simulink model "cpg_optimized"  (R2016a)
settings: Solver=FixedStepAuto  StartTime=0.0  StopTime=inf  FixedStep=0.04  RelTol=1e-3
values from neighbouring files (symbols this model uses):
  A_f = 0.1    [setup.m]
  ICNotPresent = 1    [setup.m]
  joints_in_use = [j_i_m('l_leg_hpx') j_i_m('l_leg_hpy') j_i_m('l_leg_kny') j_i_m('l_leg_aky') j_i_m('l_leg_akx') j_i_m('l_arm_shx') j_i_m('r_leg_hpx') j_i_m('r_leg_hpy') j_i_m('r_leg_kny') j_i_m('r_leg_aky') j_i_m('r_leg_akx') j_i_m('r_arm_shx')]    [setup.m]
  sigma_f = 2.2    [setup.m]
  sigma_s = 1    [setup.m]
  t_m = 0.1    [setup.m]
  t_s = 2    [setup.m]
undefined symbols (not defined in the file or in its folder): DiscIntNeverNeededParam, get, Position, SendJointCommand, SetThisJoint
libraries: fuzblock x72, dspsnks4 x4, simulink x2, robotlib x2, dspsrcs4 x1, dspindex x1, sldrtlib x1
(part 2 of 2)

== system cpg_optimized/cell_18_2 ==
  In1 : Inport
  Add : Sum  Inputs=++-
  Add1 : Sum  Inputs=-+
  Add2 : Sum  Inputs=-+
  DTI_1 : DiscreteIntegrator  InitialCondition=0.065208  InitialConditionSetting=State (most efficient)  SampleTime=-1  ICPrevOutput=DiscIntNeverNeededParam  ICPrevScaledInput=DiscIntNeverNeededParam
  DTI_2 : DiscreteIntegrator  InitialCondition=0.029689  InitialConditionSetting=State (most efficient)  SampleTime=-1  ICPrevOutput=DiscIntNeverNeededParam  ICPrevScaledInput=DiscIntNeverNeededParam
  Gain : Gain  Gain=-1/t_m
  Gain1 : Gain  Gain=1/t_s
  Gain2 : Gain  Gain=sigma_s
  Gain3 : Gain  Gain=A_f
  Gain4 : Gain  Gain=sigma_f/A_f
  Trigonometric Function : Trigonometry  Operator=tanh
  Out1 : Outport
  wires:
  Gain/1 -> DTI_1/1
  Add/1 -> Gain/1
  Gain2/1 -> Add1/2
  Gain3/1 -> Add2/1
  Add2/1 -> Add/1
  DTI_1/1 -> Out1/1, Gain2/1, Gain4/1, Add2/2  "V"
  Trigonometric Function/1 -> Gain3/1
  Gain4/1 -> Trigonometric Function/1
  In1/1 -> Add/3
  Add1/1 -> Gain1/1
  Gain1/1 -> DTI_2/1
  DTI_2/1 -> Add1/1, Add/2  "q"

== system cpg_optimized/cell_25_1 ==
  In1 : Inport
  Add : Sum  Inputs=++-
  Add1 : Sum  Inputs=-+
  Add2 : Sum  Inputs=-+
  DTI_1 : DiscreteIntegrator  InitialCondition=0.065208  InitialConditionSetting=State (most efficient)  SampleTime=-1  ICPrevOutput=DiscIntNeverNeededParam  ICPrevScaledInput=DiscIntNeverNeededParam
  DTI_2 : DiscreteIntegrator  InitialCondition=0.029689  InitialConditionSetting=State (most efficient)  SampleTime=-1  ICPrevOutput=DiscIntNeverNeededParam  ICPrevScaledInput=DiscIntNeverNeededParam
  Gain : Gain  Gain=-1/t_m
  Gain1 : Gain  Gain=1/t_s
  Gain2 : Gain  Gain=sigma_s
  Gain3 : Gain  Gain=A_f
  Gain4 : Gain  Gain=sigma_f/A_f
  Trigonometric Function : Trigonometry  Operator=tanh
  Out1 : Outport
  wires:
  Gain/1 -> DTI_1/1
  Add/1 -> Gain/1
  Gain2/1 -> Add1/2
  Gain3/1 -> Add2/1
  Add2/1 -> Add/1
  DTI_1/1 -> Out1/1, Gain2/1, Gain4/1, Add2/2  "V"
  Trigonometric Function/1 -> Gain3/1
  Gain4/1 -> Trigonometric Function/1
  In1/1 -> Add/3
  Add1/1 -> Gain1/1
  Gain1/1 -> DTI_2/1
  DTI_2/1 -> Add1/1, Add/2  "q"

== system cpg_optimized/cell_25_2 ==
  In1 : Inport
  Add : Sum  Inputs=++-
  Add1 : Sum  Inputs=-+
  Add2 : Sum  Inputs=-+
  DTI_1 : DiscreteIntegrator  InitialCondition=-0.065208  InitialConditionSetting=State (most efficient)  SampleTime=-1  ICPrevOutput=DiscIntNeverNeededParam  ICPrevScaledInput=DiscIntNeverNeededParam
  DTI_2 : DiscreteIntegrator  InitialCondition=-0.029689  InitialConditionSetting=State (most efficient)  SampleTime=-1  ICPrevOutput=DiscIntNeverNeededParam  ICPrevScaledInput=DiscIntNeverNeededParam
  Gain : Gain  Gain=-1/t_m
  Gain1 : Gain  Gain=1/t_s
  Gain2 : Gain  Gain=sigma_s
  Gain3 : Gain  Gain=A_f
  Gain4 : Gain  Gain=sigma_f/A_f
  Trigonometric Function : Trigonometry  Operator=tanh
  Out1 : Outport
  wires:
  Gain/1 -> DTI_1/1
  Add/1 -> Gain/1
  Gain2/1 -> Add1/2
  Gain3/1 -> Add2/1
  Add2/1 -> Add/1
  DTI_1/1 -> Out1/1, Gain2/1, Gain4/1, Add2/2  "V"
  Trigonometric Function/1 -> Gain3/1
  Gain4/1 -> Trigonometric Function/1
  In1/1 -> Add/3
  Add1/1 -> Gain1/1
  Gain1/1 -> DTI_2/1
  DTI_2/1 -> Add1/1, Add/2  "q"

== system cpg_optimized/cell_6_1 ==
  In1 : Inport
  Add : Sum  Inputs=++-
  Add1 : Sum  Inputs=-+
  Add2 : Sum  Inputs=-+
  DTI_1 : DiscreteIntegrator  InitialCondition=-0.059359  InitialConditionSetting=State (most efficient)  SampleTime=-1  ICPrevOutput=DiscIntNeverNeededParam  ICPrevScaledInput=DiscIntNeverNeededParam
  DTI_2 : DiscreteIntegrator  InitialCondition=-0.031714  InitialConditionSetting=State (most efficient)  SampleTime=-1  ICPrevOutput=DiscIntNeverNeededParam  ICPrevScaledInput=DiscIntNeverNeededParam
  Gain : Gain  Gain=-1/t_m
  Gain1 : Gain  Gain=1/t_s
  Gain2 : Gain  Gain=sigma_s
  Gain3 : Gain  Gain=A_f
  Gain4 : Gain  Gain=sigma_f/A_f
  Trigonometric Function : Trigonometry  Operator=tanh
  Out1 : Outport
  wires:
  Gain/1 -> DTI_1/1
  Add/1 -> Gain/1
  Gain2/1 -> Add1/2
  Gain3/1 -> Add2/1
  Add2/1 -> Add/1
  DTI_1/1 -> Out1/1, Gain2/1, Gain4/1, Add2/2  "V"
  Trigonometric Function/1 -> Gain3/1
  Gain4/1 -> Trigonometric Function/1
  In1/1 -> Add/3
  Add1/1 -> Gain1/1
  Gain1/1 -> DTI_2/1
  DTI_2/1 -> Add1/1, Add/2  "q"

== system cpg_optimized/cell_6_2 ==
  In1 : Inport
  Add : Sum  Inputs=++-
  Add1 : Sum  Inputs=-+
  Add2 : Sum  Inputs=-+
  DTI_1 : DiscreteIntegrator  InitialCondition=0.059359  InitialConditionSetting=State (most efficient)  SampleTime=-1  ICPrevOutput=DiscIntNeverNeededParam  ICPrevScaledInput=DiscIntNeverNeededParam
  DTI_2 : DiscreteIntegrator  InitialCondition=0.031714  InitialConditionSetting=State (most efficient)  SampleTime=-1  ICPrevOutput=DiscIntNeverNeededParam  ICPrevScaledInput=DiscIntNeverNeededParam
  Gain : Gain  Gain=-1/t_m
  Gain1 : Gain  Gain=1/t_s
  Gain2 : Gain  Gain=sigma_s
  Gain3 : Gain  Gain=A_f
  Gain4 : Gain  Gain=sigma_f/A_f
  Trigonometric Function : Trigonometry  Operator=tanh
  Out1 : Outport
  wires:
  Gain/1 -> DTI_1/1
  Add/1 -> Gain/1
  Gain2/1 -> Add1/2
  Gain3/1 -> Add2/1
  Add2/1 -> Add/1
  DTI_1/1 -> Out1/1, Gain2/1, Gain4/1, Add2/2  "V"
  Trigonometric Function/1 -> Gain3/1
  Gain4/1 -> Trigonometric Function/1
  In1/1 -> Add/3
  Add1/1 -> Gain1/1
  Gain1/1 -> DTI_2/1
  DTI_2/1 -> Add1/1, Add/2  "q"

== system cpg_optimized/cell_7_1 ==
  In1 : Inport
  Add : Sum  Inputs=++-
  Add1 : Sum  Inputs=-+
  Add2 : Sum  Inputs=-+
  DTI_1 : DiscreteIntegrator  InitialCondition=0.059359  InitialConditionSetting=State (most efficient)  SampleTime=-1  ICPrevOutput=DiscIntNeverNeededParam  ICPrevScaledInput=DiscIntNeverNeededParam
  DTI_2 : DiscreteIntegrator  InitialCondition=0.031714  InitialConditionSetting=State (most efficient)  SampleTime=-1  ICPrevOutput=DiscIntNeverNeededParam  ICPrevScaledInput=DiscIntNeverNeededParam
  Gain : Gain  Gain=-1/t_m
  Gain1 : Gain  Gain=1/t_s
  Gain2 : Gain  Gain=sigma_s
  Gain3 : Gain  Gain=A_f
  Gain4 : Gain  Gain=sigma_f/A_f
  Trigonometric Function : Trigonometry  Operator=tanh
  Out1 : Outport
  wires:
  Gain/1 -> DTI_1/1
  Add/1 -> Gain/1
  Gain2/1 -> Add1/2
  Gain3/1 -> Add2/1
  Add2/1 -> Add/1
  DTI_1/1 -> Out1/1, Gain2/1, Gain4/1, Add2/2  "V"
  Trigonometric Function/1 -> Gain3/1
  Gain4/1 -> Trigonometric Function/1
  In1/1 -> Add/3
  Add1/1 -> Gain1/1
  Gain1/1 -> DTI_2/1
  DTI_2/1 -> Add1/1, Add/2  "q"

== system cpg_optimized/cell_7_2 ==
  In1 : Inport
  Add : Sum  Inputs=++-
  Add1 : Sum  Inputs=-+
  Add2 : Sum  Inputs=-+
  DTI_1 : DiscreteIntegrator  InitialCondition=-0.059359  InitialConditionSetting=State (most efficient)  SampleTime=-1  ICPrevOutput=DiscIntNeverNeededParam  ICPrevScaledInput=DiscIntNeverNeededParam
  DTI_2 : DiscreteIntegrator  InitialCondition=-0.031714  InitialConditionSetting=State (most efficient)  SampleTime=-1  ICPrevOutput=DiscIntNeverNeededParam  ICPrevScaledInput=DiscIntNeverNeededParam
  Gain : Gain  Gain=-1/t_m
  Gain1 : Gain  Gain=1/t_s
  Gain2 : Gain  Gain=sigma_s
  Gain3 : Gain  Gain=A_f
  Gain4 : Gain  Gain=sigma_f/A_f
  Trigonometric Function : Trigonometry  Operator=tanh
  Out1 : Outport
  wires:
  Gain/1 -> DTI_1/1
  Add/1 -> Gain/1
  Gain2/1 -> Add1/2
  Gain3/1 -> Add2/1
  Add2/1 -> Add/1
  DTI_1/1 -> Out1/1, Gain2/1, Gain4/1, Add2/2  "V"
  Trigonometric Function/1 -> Gain3/1
  Gain4/1 -> Trigonometric Function/1
  In1/1 -> Add/3
  Add1/1 -> Gain1/1
  Gain1/1 -> DTI_2/1
  DTI_2/1 -> Add1/1, Add/2  "q"

== system cpg_optimized/cell_8_1 ==
  In1 : Inport
  Add : Sum  Inputs=++-
  Add1 : Sum  Inputs=-+
  Add2 : Sum  Inputs=-+
  DTI_1 : DiscreteIntegrator  InitialCondition=0.059359  InitialConditionSetting=State (most efficient)  SampleTime=-1  ICPrevOutput=DiscIntNeverNeededParam  ICPrevScaledInput=DiscIntNeverNeededParam
  DTI_2 : DiscreteIntegrator  InitialCondition=0.031714  InitialConditionSetting=State (most efficient)  SampleTime=-1  ICPrevOutput=DiscIntNeverNeededParam  ICPrevScaledInput=DiscIntNeverNeededParam
  Gain : Gain  Gain=-1/t_m
  Gain1 : Gain  Gain=1/t_s
  Gain2 : Gain  Gain=sigma_s
  Gain3 : Gain  Gain=A_f
  Gain4 : Gain  Gain=sigma_f/A_f
  Trigonometric Function : Trigonometry  Operator=tanh
  Out1 : Outport
  wires:
  Gain/1 -> DTI_1/1
  Add/1 -> Gain/1
  Gain2/1 -> Add1/2
  Gain3/1 -> Add2/1
  Add2/1 -> Add/1
  DTI_1/1 -> Out1/1, Gain2/1, Gain4/1, Add2/2  "V"
  Trigonometric Function/1 -> Gain3/1
  Gain4/1 -> Trigonometric Function/1
  In1/1 -> Add/3
  Add1/1 -> Gain1/1
  Gain1/1 -> DTI_2/1
  DTI_2/1 -> Add1/1, Add/2  "q"

== system cpg_optimized/cell_8_2 ==
  In1 : Inport
  Add : Sum  Inputs=++-
  Add1 : Sum  Inputs=-+
  Add2 : Sum  Inputs=-+
  DTI_1 : DiscreteIntegrator  InitialCondition=-0.059359  InitialConditionSetting=State (most efficient)  SampleTime=-1  ICPrevOutput=DiscIntNeverNeededParam  ICPrevScaledInput=DiscIntNeverNeededParam
  DTI_2 : DiscreteIntegrator  InitialCondition=-0.031714  InitialConditionSetting=State (most efficient)  SampleTime=-1  ICPrevOutput=DiscIntNeverNeededParam  ICPrevScaledInput=DiscIntNeverNeededParam
  Gain : Gain  Gain=-1/t_m
  Gain1 : Gain  Gain=1/t_s
  Gain2 : Gain  Gain=sigma_s
  Gain3 : Gain  Gain=A_f
  Gain4 : Gain  Gain=sigma_f/A_f
  Trigonometric Function : Trigonometry  Operator=tanh
  Out1 : Outport
  wires:
  Gain/1 -> DTI_1/1
  Add/1 -> Gain/1
  Gain2/1 -> Add1/2
  Gain3/1 -> Add2/1
  Add2/1 -> Add/1
  DTI_1/1 -> Out1/1, Gain2/1, Gain4/1, Add2/2  "V"
  Trigonometric Function/1 -> Gain3/1
  Gain4/1 -> Trigonometric Function/1
  In1/1 -> Add/3
  Add1/1 -> Gain1/1
  Gain1/1 -> DTI_2/1
  DTI_2/1 -> Add1/1, Add/2  "q"

== system cpg_optimized/cell_9_1 ==
  In1 : Inport
  Add : Sum  Inputs=++-
  Add1 : Sum  Inputs=-+
  Add2 : Sum  Inputs=-+
  DTI_1 : DiscreteIntegrator  InitialCondition=-0.059366  InitialConditionSetting=State (most efficient)  SampleTime=-1  ICPrevOutput=DiscIntNeverNeededParam  ICPrevScaledInput=DiscIntNeverNeededParam
  DTI_2 : DiscreteIntegrator  InitialCondition=-0.031711  InitialConditionSetting=State (most efficient)  SampleTime=-1  ICPrevOutput=DiscIntNeverNeededParam  ICPrevScaledInput=DiscIntNeverNeededParam
  Gain : Gain  Gain=-1/t_m
  Gain1 : Gain  Gain=1/t_s
  Gain2 : Gain  Gain=sigma_s
  Gain3 : Gain  Gain=A_f
  Gain4 : Gain  Gain=sigma_f/A_f
  Trigonometric Function : Trigonometry  Operator=tanh
  Out1 : Outport
  wires:
  Gain/1 -> DTI_1/1
  Add/1 -> Gain/1
  Gain2/1 -> Add1/2
  Gain3/1 -> Add2/1
  Add2/1 -> Add/1
  DTI_1/1 -> Out1/1, Gain2/1, Gain4/1, Add2/2  "V"
  Trigonometric Function/1 -> Gain3/1
  Gain4/1 -> Trigonometric Function/1
  In1/1 -> Add/3
  Add1/1 -> Gain1/1
  Gain1/1 -> DTI_2/1
  DTI_2/1 -> Add1/1, Add/2  "q"

== system cpg_optimized/cell_9_2 ==
  In1 : Inport
  Add : Sum  Inputs=++-
  Add1 : Sum  Inputs=-+
  Add2 : Sum  Inputs=-+
  DTI_1 : DiscreteIntegrator  InitialCondition=0.059366  InitialConditionSetting=State (most efficient)  SampleTime=-1  ICPrevOutput=DiscIntNeverNeededParam  ICPrevScaledInput=DiscIntNeverNeededParam
  DTI_2 : DiscreteIntegrator  InitialCondition=0.031711  InitialConditionSetting=State (most efficient)  SampleTime=-1  ICPrevOutput=DiscIntNeverNeededParam  ICPrevScaledInput=DiscIntNeverNeededParam
  Gain : Gain  Gain=-1/t_m
  Gain1 : Gain  Gain=1/t_s
  Gain2 : Gain  Gain=sigma_s
  Gain3 : Gain  Gain=A_f
  Gain4 : Gain  Gain=sigma_f/A_f
  Trigonometric Function : Trigonometry  Operator=tanh
  Out1 : Outport
  wires:
  Gain/1 -> DTI_1/1
  Add/1 -> Gain/1
  Gain2/1 -> Add1/2
  Gain3/1 -> Add2/1
  Add2/1 -> Add/1
  DTI_1/1 -> Out1/1, Gain2/1, Gain4/1, Add2/2  "V"
  Trigonometric Function/1 -> Gain3/1
  Gain4/1 -> Trigonometric Function/1
  In1/1 -> Add/3
  Add1/1 -> Gain1/1
  Gain1/1 -> DTI_2/1
  DTI_2/1 -> Add1/1, Add/2  "q"

== system cpg_optimized/AS1/If Action Subsystem1 ==
  In1 : Inport
  Action Port : ActionPort  ActionType=else
  Out1 : Outport
  wires:
  In1/1 -> Out1/1

== system cpg_optimized/AS1/If Action Subsystem3 ==
  In1 : Inport
  Action Port : ActionPort  ActionType=then
  Out1 : Outport
  wires:
  In1/1 -> Out1/1

== system cpg_optimized/AS2/If Action Subsystem1 ==
  In1 : Inport
  Action Port : ActionPort  ActionType=else
  Out1 : Outport
  wires:
  In1/1 -> Out1/1

== system cpg_optimized/AS2/If Action Subsystem3 ==
  In1 : Inport
  Action Port : ActionPort  ActionType=then
  Out1 : Outport
  wires:
  In1/1 -> Out1/1

== system cpg_optimized/PF_MN_13/If Action Subsystem ==
  In1 : Inport
  Action Port : ActionPort  ActionType=else
  Out1 : Outport
  wires:
  In1/1 -> Out1/1

== system cpg_optimized/PF_MN_13/If Action Subsystem1 ==
  In1 : Inport
  Action Port : ActionPort  ActionType=then
  Out1 : Outport
  wires:
  In1/1 -> Out1/1

== system cpg_optimized/PF_MN_7/If Action Subsystem ==
  In1 : Inport
  Action Port : ActionPort  ActionType=else
  Out1 : Outport
  wires:
  In1/1 -> Out1/1

== system cpg_optimized/PF_MN_7/If Action Subsystem1 ==
  In1 : Inport
  Action Port : ActionPort  ActionType=then
  Out1 : Outport
  wires:
  In1/1 -> Out1/1

== matlab function cpg_optimized/MATLAB Function1 ==
  data: u input
function fcn(u)
	coder.extrinsic('bdroot')
    coder.extrinsic('set_param')
    if u > 0
        set_param(bdroot,'SimulationCommand','pause')
    end
end

== matlab function cpg_optimized/MATLAB Function ==
  data: msg input; LFootX output; LFootY output; RFootX output; RFootY output
function [LFootX, LFootY, RFootX, RFootY] = fcn(msg)
%#codegen
LFootX = [0 0];
LFootY = [0 0];
RFootX = [0 0];
RFootY = [0 0];

footBF = [msg.FootBF0 msg.FootBF1];
midFoot = [msg.SdfMidFoot0 msg.SdfMidFoot1];

for i=1:length(midFoot)
    if footBF(i).Z > 800
        %Apply transform
        eul = quat2eul([midFoot(i).Orientation.X midFoot(i).Orientation.Y midFoot(i).Orientation.Z midFoot(i).Orientation.W]);
        R = rotz(eul(3));
        comCoor = (R*msg.ComEst)' - [midFoot(i).Position.X midFoot(i).Position.Y midFoot(i).Position.Z];
        
        %Determine firing region
        if i == 1
            if comCoor(1) > 0
                if comCoor(1) < 0.3
                    comCoor(1) = 0;
                else
                    comCoor(1) = comCoor(1) - 0.3;
                end
            end
        else
            if comCoor(1) < 0
                if comCoor(1) > -0.3
                    comCoor(1) = 0;
                else
                    comCoor(1) = comCoor(1) + 0.3;
                end
            end
        end
        
        if comCoor(2) > 0
            if comCoor(2) < 0.7
                comCoor(2) = 0;
            else
                comCoor(2) = comCoor(2) - 0.7;
            end
        end
        %Apply sigmoid activation
        x = 1/(1+exp(-5*comCoor(1)));
        y = 1/(1+exp(-5*comCoor(2)));
        
        if i == 1
            LFootX = [x -x];
            LFootY = [y -y];
        else
            RFootX = [x -x];
            RFootY = [y -y];
        end
    end
end
end
